simulink model "Roll_Diff_SS_D_1"  (R2013a)
settings: Solver=ode45  StartTime=0.0  StopTime=sim_length  RelTol=1e-3
values from neighbouring files (symbols this model uses):
  A_Roll_d = [1  0.03  0.0205960284122; 0  1  1.28179110803; 0  0  0.651439057531]    [Roll_Controller_SS_D_Data.mat]    (also in Roll_Controller_SS_D_Data[Conflict].mat; Roll_Controller_Sample_Time.m = A_d; State_Space_Roll_D_1.m = A_d)
  B_Roll_d = [0.00304427286801 0.294228977317 0.348560942469]    [Roll_Controller_SS_D_Data.mat]    (also in Roll_Controller_SS_D_Data[Conflict].mat; Roll_Controller_Sample_Time.m = B_d; State_Space_Roll_D_1.m = B_d)
  C_Roll_d = [1  0  0; 0  1  0]    [Roll_Controller_SS_D_Data.mat]    (also in Roll_Controller_SS_D_Data[Conflict].mat; Roll_Controller_Sample_Time.m = C_d; State_Space_Roll_D_1.m = C_d)
  Feed_Forward_Roll_d = 1/8    (= 0.125)    [Height_Controller_Sample_Time.m]    (also in Roll_Controller_SS_D_Data.mat; Roll_Controller_SS_D_Data[Conflict].mat; Roll_Controller_Sample_Time.m; State_Space_Height_D_1.m)
  G_Roll_d = [0.73387095133  0.036221570993; -0.0712605684884  1.12257105862; -0.0212805421137  0.11676537131]    [Roll_Controller_SS_D_Data.mat]    (also in Roll_Controller_SS_D_Data[Conflict].mat = [0.497083466726  0.0324399525972; -0.127651874026  0.6516223; Roll_Controller_Sample_Time.m = place(A_d',C_d',P)'; State_Space_Roll_D_1.m = place(A_d',C_d',P)')
  K_Roll_d = [1.02676834214 0.239868892992 0.659032552261]    [Roll_Controller_SS_D_Data.mat]    (also in Roll_Controller_SS_D_Data[Conflict].mat = [1.62241539227 0.326086850397 0.838371786069]; Roll_Controller_Sample_Time.m = K_Roll_Reg(1:end-1); State_Space_Roll_D_1.m = K_Roll_Reg(1:end-1))
  K_Roll_i = -1.92048833324    [Roll_Controller_SS_D_Data.mat]    (also in Roll_Controller_SS_D_Data[Conflict].mat = -1.83467215461; Roll_Controller_Sample_Time.m = K_Roll_Reg(end); State_Space_Roll_D_1.m = K_Roll_Reg(end))
  Ts = 30e-3    (= 0.03)    [All_Controller_Sample_Time.m]    (also in State_Space_Height_D_1.m = 0.02; State_Space_Roll_D_1.m = 0.02; State_Space_Yaw_D_2.m = 0.02)
undefined symbols (not defined in the file or in its folder): DiscIntNeverNeededParam, I_Theta, Kf, L, Motor_TimeConstant
settings Model: Creator=Ross  LastModifiedBy=Ross

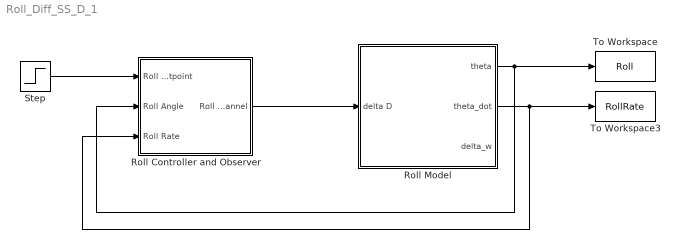
== system Roll_Diff_SS_D_1 ==
  Roll Controller and Observer : Subsystem
  Roll Model : Subsystem
  Step : Step  SampleTime=0
  To Workspace : ToWorkspace  VariableName=Roll  SampleTime=-1  SaveFormat=Timeseries
  To Workspace3 : ToWorkspace  VariableName=RollRate  SampleTime=-1  SaveFormat=Timeseries
  wires:
  Roll Model/1(theta) -> Roll Controller and Observer/2(Roll Angle), To Workspace/1
  Roll Model/2(theta_dot) -> Roll Controller and Observer/3(Roll Rate), To Workspace3/1
  Step/1 -> Roll Controller and Observer/1(Roll Setpoint)
  Roll Controller and Observer/1(Roll Channel) -> Roll Model/1(delta D)

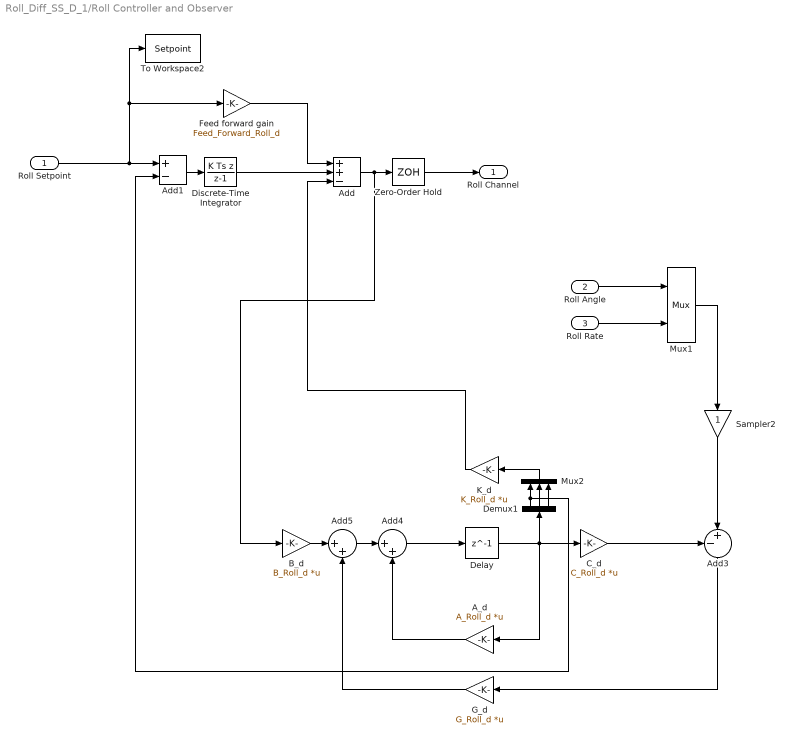
== system Roll_Diff_SS_D_1/Roll Controller and Observer ==
  Roll Setpoint : Inport
  Roll Angle : Inport  Port=2
  Roll Rate : Inport  Port=3
  A_d : Gain  Gain=A_Roll_d  Multiplication=Matrix(K*u)  SampleTime=Ts
  Add : Sum  Inputs=++-
  Add1 : Sum  Inputs=+-
  Add3 : Sum  Inputs=-+|
  Add4 : Sum  Inputs=|++
  Add5 : Sum  Inputs=|++
  "B_d " : Gain  Gain=B_Roll_d  Multiplication=Matrix(K*u)  SampleTime=Ts
  "C_d " : Gain  Gain=C_Roll_d  Multiplication=Matrix(K*u)  SampleTime=Ts
  Delay : Delay  DelayLength=1  InitialCondition=0  SampleTime=Ts
  Demux1 : Demux  Outputs=3
  Discrete-Time Integrator : DiscreteIntegrator  IntegratorMethod=Integration: Backward Euler  gainval=-K_Roll_i  SampleTime=Ts  ICPrevOutput=DiscIntNeverNeededParam  ICPrevScaledInput=DiscIntNeverNeededParam
  Feed forward gain : Gain  Gain=Feed_Forward_Roll_d  SampleTime=Ts
  G_d : Gain  Gain=G_Roll_d  Multiplication=Matrix(K*u)  SampleTime=Ts
  K_d : Gain  Gain=K_Roll_d  Multiplication=Matrix(K*u)  SampleTime=Ts
  Mux1 : Mux  Inputs=2
      settings: DisplayOption=signals
  Mux2 : Mux  Inputs=3
  Sampler2 : Gain  SampleTime=Ts
  To Workspace2 : ToWorkspace  VariableName=Setpoint  SampleTime=-1  SaveFormat=Timeseries
  Zero-Order Hold : ZeroOrderHold  SampleTime=Ts
  Roll Channel : Outport
  wires:
  Roll Rate/1 -> Mux1/2
  Roll Angle/1 -> Mux1/1
  Add5/1 -> Add4/1
  Demux1/3 -> Mux2/3
  Mux1/1 -> Sampler2/1
  G_d/1 -> Add5/2
  Demux1/2 -> Mux2/2
  A_d/1 -> Add4/2
  Add4/1 -> Delay/1
  "C_d "/1 -> Add3/1
  K_d/1 -> Add/3
  Sampler2/1 -> Add3/2
  Add/1 -> "B_d "/1, Zero-Order Hold/1
  "B_d "/1 -> Add5/1
  Demux1/1 -> Add1/2, Mux2/1
  Mux2/1 -> K_d/1
  Add3/1 -> G_d/1
  Delay/1 -> "C_d "/1, Demux1/1, A_d/1
  Zero-Order Hold/1 -> Roll Channel/1
  Discrete-Time Integrator/1 -> Add/2
  Roll Setpoint/1 -> To Workspace2/1, Feed forward gain/1, Add1/1
  Add1/1 -> Discrete-Time Integrator/1
  Feed forward gain/1 -> Add/1

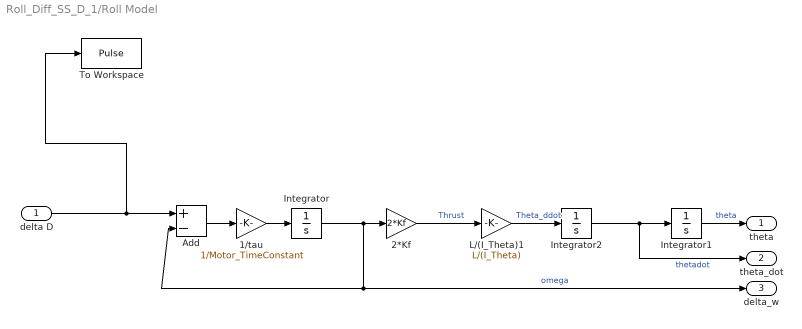
== system Roll_Diff_SS_D_1/Roll Model ==
  delta D : Inport
  1/tau : Gain  Gain=1/Motor_TimeConstant
  2*Kf : Gain  Gain=2*Kf
  Add : Sum  Inputs=+-
  Integrator : Integrator
  Integrator1 : Integrator
  Integrator2 : Integrator
  L/(I_Theta)1 : Gain  Gain=L/(I_Theta)
  To Workspace : ToWorkspace  VariableName=Pulse  SampleTime=-1  SaveFormat=Timeseries
  theta : Outport
  theta_dot : Outport  Port=2
  delta_w : Outport  Port=3
  wires:
  2*Kf/1 -> L/(I_Theta)1/1  "Thrust"
  Integrator2/1 -> theta_dot/1, Integrator1/1  "thetadot"
  Add/1 -> 1/tau/1
  delta D/1 -> To Workspace/1, Add/1
  Integrator/1 -> 2*Kf/1, Add/2, delta_w/1  "omega"
  1/tau/1 -> Integrator/1
  Integrator1/1 -> theta/1  "theta"
  L/(I_Theta)1/1 -> Integrator2/1  "Theta_ddot"
